simulink model "xieboduoji_13fangzhennow"  (R2023a)
settings: Solver=ode4  StartTime=0.0  StopTime=2.2  FixedStep=5e-7  RelTol=1e-3
undefined symbols (not defined in the file or in its folder): magnitude
libraries: simulink x417, spsRMSLib x70, spsCurrentMeasurementLib x32, spsVoltageMeasurementLib x31, powerlib_meascontrol x24, spsFourierLib x21, spsGroundLib x19, spsThreePhasePISectionLineLib x17, spsThreePhaseSeriesRLCBranchLib x14, spsdq0toAlphaBetaZeroLib x13, spsSeriesRLCBranchLib x11, spsUniversalBridgeLib x11
(part 8 of 12)

== system xieboduoji_13fangzhennow/node3/谐波源/Subsystem1/RMS1 ==
  u1 : Inport
  u3 : Inport  Port=2
  u4 : Inport  Port=3
  u5 : Inport  Port=4
  u6 : Inport  Port=5
  u2 : Inport  Port=6
  Trigger : TriggerPort  VariantControl=(inherit)
  Scope : Scope  Commented=on
  Scope1 : Scope  Commented=on
  xunidiandao : MATLAB Function  TreatAsAtomicUnit=on
  k1 : Outport  VectorParamsAs1DForOutWhenUnconnected=off
  k2 : Outport  Port=2  VectorParamsAs1DForOutWhenUnconnected=off
  k3 : Outport  Port=3  VectorParamsAs1DForOutWhenUnconnected=off
  k4 : Outport  Port=4  VectorParamsAs1DForOutWhenUnconnected=off
  k5 : Outport  Port=5  VectorParamsAs1DForOutWhenUnconnected=off
  k6 : Outport  Port=6  VectorParamsAs1DForOutWhenUnconnected=off
  k7 : Outport  Port=7  VectorParamsAs1DForOutWhenUnconnected=off
  k8 : Outport  Port=8  VectorParamsAs1DForOutWhenUnconnected=off
  k9 : Outport  Port=9  VectorParamsAs1DForOutWhenUnconnected=off
  k10 : Outport  Port=10  VectorParamsAs1DForOutWhenUnconnected=off
  k11 : Outport  Port=11  VectorParamsAs1DForOutWhenUnconnected=off
  k12 : Outport  Port=12  VectorParamsAs1DForOutWhenUnconnected=off
  wires:
  xunidiandao/13(x) -> Scope/1
  u3/1 -> xunidiandao/2(u2)
  u4/1 -> xunidiandao/3(u3)
  u5/1 -> xunidiandao/4(u4)
  u6/1 -> xunidiandao/5(u5)
  u2/1 -> xunidiandao/6(u6)
  u1/1 -> xunidiandao/1(u1)
  xunidiandao/12(y66) -> k12/1
  xunidiandao/11(y6) -> k11/1
  xunidiandao/10(y55) -> k10/1
  xunidiandao/9(y5) -> k9/1
  xunidiandao/8(y44) -> k8/1
  xunidiandao/7(y4) -> k7/1
  xunidiandao/6(y33) -> k6/1
  xunidiandao/5(y3) -> k5/1
  xunidiandao/4(y22) -> k4/1
  xunidiandao/3(y2) -> k3/1
  xunidiandao/2(y11) -> k2/1
  xunidiandao/1(y1) -> k1/1, Scope1/1

== system xieboduoji_13fangzhennow/node3/谐波源/Subsystem2/RMS1 ==
  u1 : Inport
  u3 : Inport  Port=2
  u4 : Inport  Port=3
  u5 : Inport  Port=4
  u6 : Inport  Port=5
  u2 : Inport  Port=6
  Trigger : TriggerPort  VariantControl=(inherit)
  Scope : Scope  Commented=on
  Scope1 : Scope  Commented=on
  xunidiandao : MATLAB Function  TreatAsAtomicUnit=on
  k1 : Outport  VectorParamsAs1DForOutWhenUnconnected=off
  k2 : Outport  Port=2  VectorParamsAs1DForOutWhenUnconnected=off
  k3 : Outport  Port=3  VectorParamsAs1DForOutWhenUnconnected=off
  k4 : Outport  Port=4  VectorParamsAs1DForOutWhenUnconnected=off
  k5 : Outport  Port=5  VectorParamsAs1DForOutWhenUnconnected=off
  k6 : Outport  Port=6  VectorParamsAs1DForOutWhenUnconnected=off
  k7 : Outport  Port=7  VectorParamsAs1DForOutWhenUnconnected=off
  k8 : Outport  Port=8  VectorParamsAs1DForOutWhenUnconnected=off
  k9 : Outport  Port=9  VectorParamsAs1DForOutWhenUnconnected=off
  k10 : Outport  Port=10  VectorParamsAs1DForOutWhenUnconnected=off
  k11 : Outport  Port=11  VectorParamsAs1DForOutWhenUnconnected=off
  k12 : Outport  Port=12  VectorParamsAs1DForOutWhenUnconnected=off
  wires:
  xunidiandao/1(y1) -> Scope1/1, k1/1
  xunidiandao/2(y11) -> k2/1
  xunidiandao/3(y2) -> k3/1
  xunidiandao/4(y22) -> k4/1
  xunidiandao/5(y3) -> k5/1
  xunidiandao/6(y33) -> k6/1
  xunidiandao/7(y4) -> k7/1
  xunidiandao/8(y44) -> k8/1
  xunidiandao/9(y5) -> k9/1
  xunidiandao/10(y55) -> k10/1
  xunidiandao/11(y6) -> k11/1
  xunidiandao/12(y66) -> k12/1
  u1/1 -> xunidiandao/1(u1)
  u2/1 -> xunidiandao/6(u6)
  u6/1 -> xunidiandao/5(u5)
  u5/1 -> xunidiandao/4(u4)
  u4/1 -> xunidiandao/3(u3)
  u3/1 -> xunidiandao/2(u2)
  xunidiandao/13(x) -> Scope/1

== system xieboduoji_13fangzhennow/node4/谐波源/Subsystem1/RMS1 ==
  u1 : Inport
  u3 : Inport  Port=2
  u4 : Inport  Port=3
  u5 : Inport  Port=4
  u6 : Inport  Port=5
  u2 : Inport  Port=6
  Trigger : TriggerPort  VariantControl=(inherit)
  Scope : Scope  Commented=on
  Scope1 : Scope  Commented=on
  xunidiandao : MATLAB Function  TreatAsAtomicUnit=on
  k1 : Outport  VectorParamsAs1DForOutWhenUnconnected=off
  k2 : Outport  Port=2  VectorParamsAs1DForOutWhenUnconnected=off
  k3 : Outport  Port=3  VectorParamsAs1DForOutWhenUnconnected=off
  k4 : Outport  Port=4  VectorParamsAs1DForOutWhenUnconnected=off
  k5 : Outport  Port=5  VectorParamsAs1DForOutWhenUnconnected=off
  k6 : Outport  Port=6  VectorParamsAs1DForOutWhenUnconnected=off
  k7 : Outport  Port=7  VectorParamsAs1DForOutWhenUnconnected=off
  k8 : Outport  Port=8  VectorParamsAs1DForOutWhenUnconnected=off
  k9 : Outport  Port=9  VectorParamsAs1DForOutWhenUnconnected=off
  k10 : Outport  Port=10  VectorParamsAs1DForOutWhenUnconnected=off
  k11 : Outport  Port=11  VectorParamsAs1DForOutWhenUnconnected=off
  k12 : Outport  Port=12  VectorParamsAs1DForOutWhenUnconnected=off
  wires:
  xunidiandao/13(x) -> Scope/1
  u3/1 -> xunidiandao/2(u2)
  u4/1 -> xunidiandao/3(u3)
  u5/1 -> xunidiandao/4(u4)
  u6/1 -> xunidiandao/5(u5)
  u2/1 -> xunidiandao/6(u6)
  u1/1 -> xunidiandao/1(u1)
  xunidiandao/12(y66) -> k12/1
  xunidiandao/11(y6) -> k11/1
  xunidiandao/10(y55) -> k10/1
  xunidiandao/9(y5) -> k9/1
  xunidiandao/8(y44) -> k8/1
  xunidiandao/7(y4) -> k7/1
  xunidiandao/6(y33) -> k6/1
  xunidiandao/5(y3) -> k5/1
  xunidiandao/4(y22) -> k4/1
  xunidiandao/3(y2) -> k3/1
  xunidiandao/2(y11) -> k2/1
  xunidiandao/1(y1) -> k1/1, Scope1/1

== system xieboduoji_13fangzhennow/node4/谐波源/Subsystem2/RMS1 ==
  u1 : Inport
  u3 : Inport  Port=2
  u4 : Inport  Port=3
  u5 : Inport  Port=4
  u6 : Inport  Port=5
  u2 : Inport  Port=6
  Trigger : TriggerPort  VariantControl=(inherit)
  Scope : Scope  Commented=on
  Scope1 : Scope  Commented=on
  xunidiandao : MATLAB Function  TreatAsAtomicUnit=on
  k1 : Outport  VectorParamsAs1DForOutWhenUnconnected=off
  k2 : Outport  Port=2  VectorParamsAs1DForOutWhenUnconnected=off
  k3 : Outport  Port=3  VectorParamsAs1DForOutWhenUnconnected=off
  k4 : Outport  Port=4  VectorParamsAs1DForOutWhenUnconnected=off
  k5 : Outport  Port=5  VectorParamsAs1DForOutWhenUnconnected=off
  k6 : Outport  Port=6  VectorParamsAs1DForOutWhenUnconnected=off
  k7 : Outport  Port=7  VectorParamsAs1DForOutWhenUnconnected=off
  k8 : Outport  Port=8  VectorParamsAs1DForOutWhenUnconnected=off
  k9 : Outport  Port=9  VectorParamsAs1DForOutWhenUnconnected=off
  k10 : Outport  Port=10  VectorParamsAs1DForOutWhenUnconnected=off
  k11 : Outport  Port=11  VectorParamsAs1DForOutWhenUnconnected=off
  k12 : Outport  Port=12  VectorParamsAs1DForOutWhenUnconnected=off
  wires:
  xunidiandao/1(y1) -> Scope1/1, k1/1
  xunidiandao/2(y11) -> k2/1
  xunidiandao/3(y2) -> k3/1
  xunidiandao/4(y22) -> k4/1
  xunidiandao/5(y3) -> k5/1
  xunidiandao/6(y33) -> k6/1
  xunidiandao/7(y4) -> k7/1
  xunidiandao/8(y44) -> k8/1
  xunidiandao/9(y5) -> k9/1
  xunidiandao/10(y55) -> k10/1
  xunidiandao/11(y6) -> k11/1
  xunidiandao/12(y66) -> k12/1
  u1/1 -> xunidiandao/1(u1)
  u2/1 -> xunidiandao/6(u6)
  u6/1 -> xunidiandao/5(u5)
  u5/1 -> xunidiandao/4(u4)
  u4/1 -> xunidiandao/3(u3)
  u3/1 -> xunidiandao/2(u2)
  xunidiandao/13(x) -> Scope/1

== system xieboduoji_13fangzhennow/node5/谐波源/Subsystem1/RMS1 ==
  u1 : Inport
  u3 : Inport  Port=2
  u4 : Inport  Port=3
  u5 : Inport  Port=4
  u6 : Inport  Port=5
  u2 : Inport  Port=6
  Trigger : TriggerPort  VariantControl=(inherit)
  Scope : Scope  Commented=on
  Scope1 : Scope  Commented=on
  xunidiandao : MATLAB Function  TreatAsAtomicUnit=on
  k1 : Outport  VectorParamsAs1DForOutWhenUnconnected=off
  k2 : Outport  Port=2  VectorParamsAs1DForOutWhenUnconnected=off
  k3 : Outport  Port=3  VectorParamsAs1DForOutWhenUnconnected=off
  k4 : Outport  Port=4  VectorParamsAs1DForOutWhenUnconnected=off
  k5 : Outport  Port=5  VectorParamsAs1DForOutWhenUnconnected=off
  k6 : Outport  Port=6  VectorParamsAs1DForOutWhenUnconnected=off
  k7 : Outport  Port=7  VectorParamsAs1DForOutWhenUnconnected=off
  k8 : Outport  Port=8  VectorParamsAs1DForOutWhenUnconnected=off
  k9 : Outport  Port=9  VectorParamsAs1DForOutWhenUnconnected=off
  k10 : Outport  Port=10  VectorParamsAs1DForOutWhenUnconnected=off
  k11 : Outport  Port=11  VectorParamsAs1DForOutWhenUnconnected=off
  k12 : Outport  Port=12  VectorParamsAs1DForOutWhenUnconnected=off
  wires:
  xunidiandao/13(x) -> Scope/1
  u3/1 -> xunidiandao/2(u2)
  u4/1 -> xunidiandao/3(u3)
  u5/1 -> xunidiandao/4(u4)
  u6/1 -> xunidiandao/5(u5)
  u2/1 -> xunidiandao/6(u6)
  u1/1 -> xunidiandao/1(u1)
  xunidiandao/12(y66) -> k12/1
  xunidiandao/11(y6) -> k11/1
  xunidiandao/10(y55) -> k10/1
  xunidiandao/9(y5) -> k9/1
  xunidiandao/8(y44) -> k8/1
  xunidiandao/7(y4) -> k7/1
  xunidiandao/6(y33) -> k6/1
  xunidiandao/5(y3) -> k5/1
  xunidiandao/4(y22) -> k4/1
  xunidiandao/3(y2) -> k3/1
  xunidiandao/2(y11) -> k2/1
  xunidiandao/1(y1) -> k1/1, Scope1/1

== system xieboduoji_13fangzhennow/node5/谐波源/Subsystem2/RMS1 ==
  u1 : Inport
  u3 : Inport  Port=2
  u4 : Inport  Port=3
  u5 : Inport  Port=4
  u6 : Inport  Port=5
  u2 : Inport  Port=6
  Trigger : TriggerPort  VariantControl=(inherit)
  Scope : Scope  Commented=on
  Scope1 : Scope  Commented=on
  xunidiandao : MATLAB Function  TreatAsAtomicUnit=on
  k1 : Outport  VectorParamsAs1DForOutWhenUnconnected=off
  k2 : Outport  Port=2  VectorParamsAs1DForOutWhenUnconnected=off
  k3 : Outport  Port=3  VectorParamsAs1DForOutWhenUnconnected=off
  k4 : Outport  Port=4  VectorParamsAs1DForOutWhenUnconnected=off
  k5 : Outport  Port=5  VectorParamsAs1DForOutWhenUnconnected=off
  k6 : Outport  Port=6  VectorParamsAs1DForOutWhenUnconnected=off
  k7 : Outport  Port=7  VectorParamsAs1DForOutWhenUnconnected=off
  k8 : Outport  Port=8  VectorParamsAs1DForOutWhenUnconnected=off
  k9 : Outport  Port=9  VectorParamsAs1DForOutWhenUnconnected=off
  k10 : Outport  Port=10  VectorParamsAs1DForOutWhenUnconnected=off
  k11 : Outport  Port=11  VectorParamsAs1DForOutWhenUnconnected=off
  k12 : Outport  Port=12  VectorParamsAs1DForOutWhenUnconnected=off
  wires:
  xunidiandao/1(y1) -> Scope1/1, k1/1
  xunidiandao/2(y11) -> k2/1
  xunidiandao/3(y2) -> k3/1
  xunidiandao/4(y22) -> k4/1
  xunidiandao/5(y3) -> k5/1
  xunidiandao/6(y33) -> k6/1
  xunidiandao/7(y4) -> k7/1
  xunidiandao/8(y44) -> k8/1
  xunidiandao/9(y5) -> k9/1
  xunidiandao/10(y55) -> k10/1
  xunidiandao/11(y6) -> k11/1
  xunidiandao/12(y66) -> k12/1
  u1/1 -> xunidiandao/1(u1)
  u2/1 -> xunidiandao/6(u6)
  u6/1 -> xunidiandao/5(u5)
  u5/1 -> xunidiandao/4(u4)
  u4/1 -> xunidiandao/3(u3)
  u3/1 -> xunidiandao/2(u2)
  xunidiandao/13(x) -> Scope/1

== system xieboduoji_13fangzhennow/node8/谐波源/Subsystem1/RMS1 ==
  u1 : Inport
  u3 : Inport  Port=2
  u4 : Inport  Port=3
  u5 : Inport  Port=4
  u6 : Inport  Port=5
  u2 : Inport  Port=6
  Trigger : TriggerPort  VariantControl=(inherit)
  Scope : Scope  Commented=on
  Scope1 : Scope  Commented=on
  xunidiandao : MATLAB Function  TreatAsAtomicUnit=on
  k1 : Outport  VectorParamsAs1DForOutWhenUnconnected=off
  k2 : Outport  Port=2  VectorParamsAs1DForOutWhenUnconnected=off
  k3 : Outport  Port=3  VectorParamsAs1DForOutWhenUnconnected=off
  k4 : Outport  Port=4  VectorParamsAs1DForOutWhenUnconnected=off
  k5 : Outport  Port=5  VectorParamsAs1DForOutWhenUnconnected=off
  k6 : Outport  Port=6  VectorParamsAs1DForOutWhenUnconnected=off
  k7 : Outport  Port=7  VectorParamsAs1DForOutWhenUnconnected=off
  k8 : Outport  Port=8  VectorParamsAs1DForOutWhenUnconnected=off
  k9 : Outport  Port=9  VectorParamsAs1DForOutWhenUnconnected=off
  k10 : Outport  Port=10  VectorParamsAs1DForOutWhenUnconnected=off
  k11 : Outport  Port=11  VectorParamsAs1DForOutWhenUnconnected=off
  k12 : Outport  Port=12  VectorParamsAs1DForOutWhenUnconnected=off
  wires:
  xunidiandao/13(x) -> Scope/1
  u3/1 -> xunidiandao/2(u2)
  u4/1 -> xunidiandao/3(u3)
  u5/1 -> xunidiandao/4(u4)
  u6/1 -> xunidiandao/5(u5)
  u2/1 -> xunidiandao/6(u6)
  u1/1 -> xunidiandao/1(u1)
  xunidiandao/12(y66) -> k12/1
  xunidiandao/11(y6) -> k11/1
  xunidiandao/10(y55) -> k10/1
  xunidiandao/9(y5) -> k9/1
  xunidiandao/8(y44) -> k8/1
  xunidiandao/7(y4) -> k7/1
  xunidiandao/6(y33) -> k6/1
  xunidiandao/5(y3) -> k5/1
  xunidiandao/4(y22) -> k4/1
  xunidiandao/3(y2) -> k3/1
  xunidiandao/2(y11) -> k2/1
  xunidiandao/1(y1) -> k1/1, Scope1/1

== system xieboduoji_13fangzhennow/node8/谐波源/Subsystem2/RMS1 ==
  u1 : Inport
  u3 : Inport  Port=2
  u4 : Inport  Port=3
  u5 : Inport  Port=4
  u6 : Inport  Port=5
  u2 : Inport  Port=6
  Trigger : TriggerPort  VariantControl=(inherit)
  Scope : Scope  Commented=on
  Scope1 : Scope  Commented=on
  xunidiandao : MATLAB Function  TreatAsAtomicUnit=on
  k1 : Outport  VectorParamsAs1DForOutWhenUnconnected=off
  k2 : Outport  Port=2  VectorParamsAs1DForOutWhenUnconnected=off
  k3 : Outport  Port=3  VectorParamsAs1DForOutWhenUnconnected=off
  k4 : Outport  Port=4  VectorParamsAs1DForOutWhenUnconnected=off
  k5 : Outport  Port=5  VectorParamsAs1DForOutWhenUnconnected=off
  k6 : Outport  Port=6  VectorParamsAs1DForOutWhenUnconnected=off
  k7 : Outport  Port=7  VectorParamsAs1DForOutWhenUnconnected=off
  k8 : Outport  Port=8  VectorParamsAs1DForOutWhenUnconnected=off
  k9 : Outport  Port=9  VectorParamsAs1DForOutWhenUnconnected=off
  k10 : Outport  Port=10  VectorParamsAs1DForOutWhenUnconnected=off
  k11 : Outport  Port=11  VectorParamsAs1DForOutWhenUnconnected=off
  k12 : Outport  Port=12  VectorParamsAs1DForOutWhenUnconnected=off
  wires:
  xunidiandao/1(y1) -> Scope1/1, k1/1
  xunidiandao/2(y11) -> k2/1
  xunidiandao/3(y2) -> k3/1
  xunidiandao/4(y22) -> k4/1
  xunidiandao/5(y3) -> k5/1
  xunidiandao/6(y33) -> k6/1
  xunidiandao/7(y4) -> k7/1
  xunidiandao/8(y44) -> k8/1
  xunidiandao/9(y5) -> k9/1
  xunidiandao/10(y55) -> k10/1
  xunidiandao/11(y6) -> k11/1
  xunidiandao/12(y66) -> k12/1
  u1/1 -> xunidiandao/1(u1)
  u2/1 -> xunidiandao/6(u6)
  u6/1 -> xunidiandao/5(u5)
  u5/1 -> xunidiandao/4(u4)
  u4/1 -> xunidiandao/3(u3)
  u3/1 -> xunidiandao/2(u2)
  xunidiandao/13(x) -> Scope/1

== system xieboduoji_13fangzhennow/node12/PV15kW3/谐波检测/Subsystem/Sub ==
  In1 : Inport
  Constant1 : Constant  Value=-60*pi/180
  Constant{10,12,15,17} (4 alike) : Constant  Value=100*pi
  Constant11 : Constant  Value=5
  Constant2 : Constant  Value=-60*pi/180
  Cos : Trigonometry  Operator=cos
  Cos1 : Trigonometry  Operator=cos
  Cos2 : Trigonometry
  Cos3 : Trigonometry
  Delay : Delay  DelayLength=400  SampleTime=5e-5
  Delay1 : Delay  DelayLength=1  SampleTime=5e-5
  Delay2 : Delay  DelayLength=1  SampleTime=5e-5
  Divide{,1..3} (4 alike) : Product  Inputs=***
  Dot Product{,1..2,4} (4 alike) : DotProduct  OutDataTypeStr=Inherit: Inherit via internal rule
  Gain : Gain  Gain=2/400
  Gain10 : Gain  Gain=2/400
  Ramp{,1..3} (4 alike) : simulink/Sources/Ramp  slope=1  start=0  InitialOutput=0
  Sum{,1,3,9,18} (5 alike) : Sum  Inputs=|++
  Sum2 : Sum  Inputs=-+|
  u1 : Outport
  wires:
  [thk] -> Divide/1
  Constant11/1 -> [thk]
  Sum9/1 -> u1/1
  Dot Product1/1 -> Sum9/1
  Gain/1 -> Sum3/1
  Ramp2/1 -> Divide2/3
  Constant10/1 -> Divide/2
  Delay2/1 -> Sum18/2
  Gain10/1 -> Sum18/1
  Sum3/1 -> Delay1/1, Dot Product1/2
  Delay/1 -> Sum2/1
  Ramp1/1 -> Divide1/3
  Constant12/1 -> Divide1/2
  Divide2/1 -> Cos2/1
  Cos3/1 -> Dot Product4/2
  Dot Product2/1 -> Gain10/1
  Cos2/1 -> Dot Product2/2
  Delay1/1 -> Sum3/2
  Ramp3/1 -> Divide3/3
  [thk] -> Divide1/1
  Dot Product4/1 -> Sum9/2
  [thk] -> Divide2/1
  [thk] -> Divide3/1
  Sum18/1 -> Delay2/1, Dot Product4/1
  Constant15/1 -> Divide2/2
  In1/1 -> Sum2/2, Delay/1
  Dot Product/1 -> Gain/1
  Cos/1 -> Dot Product/1
  Divide/1 -> Cos/1
  Sum2/1 -> Dot Product/2, Dot Product2/1
  Ramp/1 -> Divide/3
  Constant17/1 -> Divide3/2
  Cos1/1 -> Dot Product1/1
  Divide1/1 -> Sum/1
  Sum/1 -> Cos1/1
  Sum1/1 -> Cos3/1
  Divide3/1 -> Sum1/1

== system xieboduoji_13fangzhennow/node12/PV15kW3/谐波检测/Subsystem/Sub1 ==
  In1 : Inport
  Constant1 : Constant  Value=-60*pi/180
  Constant{10,12,15,17} (4 alike) : Constant  Value=100*pi
  Constant11 : Constant  Value=7
  Constant2 : Constant  Value=-60*pi/180
  Cos : Trigonometry  Operator=cos
  Cos1 : Trigonometry  Operator=cos
  Cos2 : Trigonometry
  Cos3 : Trigonometry
  Delay : Delay  DelayLength=400  SampleTime=5e-5
  Delay1 : Delay  DelayLength=1  SampleTime=5e-5
  Delay2 : Delay  DelayLength=1  SampleTime=5e-5
  Divide{,1..3} (4 alike) : Product  Inputs=***
  Dot Product{,1..2,4} (4 alike) : DotProduct  OutDataTypeStr=Inherit: Inherit via internal rule
  Gain : Gain  Gain=2/400
  Gain10 : Gain  Gain=2/400
  Ramp{,1..3} (4 alike) : simulink/Sources/Ramp  slope=1  start=0  InitialOutput=0
  Sum{,1,3,9,18} (5 alike) : Sum  Inputs=|++
  Sum2 : Sum  Inputs=-+|
  u1 : Outport
  wires:
  Divide3/1 -> Sum1/1
  Sum1/1 -> Cos3/1
  Sum/1 -> Cos1/1
  Divide1/1 -> Sum/1
  Cos1/1 -> Dot Product1/1
  Constant17/1 -> Divide3/2
  Ramp/1 -> Divide/3
  Sum2/1 -> Dot Product2/1, Dot Product/2
  Divide/1 -> Cos/1
  Cos/1 -> Dot Product/1
  Dot Product/1 -> Gain/1
  In1/1 -> Delay/1, Sum2/2
  Constant15/1 -> Divide2/2
  Sum18/1 -> Dot Product4/1, Delay2/1
  [thk] -> Divide3/1
  [thk] -> Divide2/1
  Dot Product4/1 -> Sum9/2
  [thk] -> Divide1/1
  Ramp3/1 -> Divide3/3
  Delay1/1 -> Sum3/2
  Cos2/1 -> Dot Product2/2
  Dot Product2/1 -> Gain10/1
  Cos3/1 -> Dot Product4/2
  Divide2/1 -> Cos2/1
  Constant12/1 -> Divide1/2
  Ramp1/1 -> Divide1/3
  Delay/1 -> Sum2/1
  Sum3/1 -> Dot Product1/2, Delay1/1
  Gain10/1 -> Sum18/1
  Delay2/1 -> Sum18/2
  Constant10/1 -> Divide/2
  Ramp2/1 -> Divide2/3
  Gain/1 -> Sum3/1
  Dot Product1/1 -> Sum9/1
  Sum9/1 -> u1/1
  Constant11/1 -> [thk]
  [thk] -> Divide/1

== system xieboduoji_13fangzhennow/node12/PV15kW3/谐波检测/Subsystem/Sub10 ==
  In1 : Inport
  Constant1 : Constant  Value=10*pi/180
  Constant{10,12,15,17} (4 alike) : Constant  Value=100*pi
  Constant11 : Constant  Value=19
  Constant2 : Constant  Value=10*pi/180
  Cos : Trigonometry  Operator=cos
  Cos1 : Trigonometry  Operator=cos
  Cos2 : Trigonometry
  Cos3 : Trigonometry
  Delay : Delay  DelayLength=400  SampleTime=5e-5
  Delay1 : Delay  DelayLength=1  SampleTime=5e-5
  Delay2 : Delay  DelayLength=1  SampleTime=5e-5
  Divide{,1..3} (4 alike) : Product  Inputs=***
  Dot Product{,1..2,4} (4 alike) : DotProduct  OutDataTypeStr=Inherit: Inherit via internal rule
  Gain : Gain  Gain=2/400
  Gain10 : Gain  Gain=2/400
  Ramp{,1..3} (4 alike) : simulink/Sources/Ramp  slope=1  start=0  InitialOutput=0
  Sum{,1,3,9,18} (5 alike) : Sum  Inputs=|++
  Sum2 : Sum  Inputs=-+|
  u9 : Outport
  wires:
  [thk] -> Divide/1
  Constant11/1 -> [thk]
  Sum9/1 -> u9/1
  Dot Product1/1 -> Sum9/1
  Gain/1 -> Sum3/1
  Ramp2/1 -> Divide2/3
  Constant10/1 -> Divide/2
  Delay2/1 -> Sum18/2
  Gain10/1 -> Sum18/1
  Sum3/1 -> Delay1/1, Dot Product1/2
  Delay/1 -> Sum2/1
  Ramp1/1 -> Divide1/3
  Constant12/1 -> Divide1/2
  Divide2/1 -> Cos2/1
  Cos3/1 -> Dot Product4/2
  Dot Product2/1 -> Gain10/1
  Cos2/1 -> Dot Product2/2
  Delay1/1 -> Sum3/2
  Ramp3/1 -> Divide3/3
  [thk] -> Divide1/1
  Dot Product4/1 -> Sum9/2
  [thk] -> Divide2/1
  [thk] -> Divide3/1
  Sum18/1 -> Delay2/1, Dot Product4/1
  Constant15/1 -> Divide2/2
  In1/1 -> Sum2/2, Delay/1
  Cos1/1 -> Dot Product1/1
  Dot Product/1 -> Gain/1
  Cos/1 -> Dot Product/1
  Divide/1 -> Cos/1
  Sum2/1 -> Dot Product/2, Dot Product2/1
  Ramp/1 -> Divide/3
  Constant17/1 -> Divide3/2
  Divide1/1 -> Sum/1
  Sum/1 -> Cos1/1
  Divide3/1 -> Sum1/1
  Sum1/1 -> Cos3/1
  Constant2/1 -> Sum/2
  Constant1/1 -> Sum1/2

== system xieboduoji_13fangzhennow/node12/PV15kW3/谐波检测/Subsystem/Sub12 ==
  In1 : Inport
  Constant1 : Constant  Value=10*pi/180
  Constant{10,12,15,17} (4 alike) : Constant  Value=100*pi
  Constant11 : Constant  Value=17
  Constant2 : Constant  Value=10*pi/180
  Cos : Trigonometry  Operator=cos
  Cos1 : Trigonometry  Operator=cos
  Cos2 : Trigonometry
  Cos3 : Trigonometry
  Delay : Delay  DelayLength=400  SampleTime=5e-5
  Delay1 : Delay  DelayLength=1  SampleTime=5e-5
  Delay2 : Delay  DelayLength=1  SampleTime=5e-5
  Divide{,1..3} (4 alike) : Product  Inputs=***
  Dot Product{,1..2,4} (4 alike) : DotProduct  OutDataTypeStr=Inherit: Inherit via internal rule
  Gain : Gain  Gain=2/400
  Gain10 : Gain  Gain=2/400
  Ramp{,1..3} (4 alike) : simulink/Sources/Ramp  slope=1  start=0  InitialOutput=0
  Sum{,1,3,9,18} (5 alike) : Sum  Inputs=|++
  Sum2 : Sum  Inputs=-+|
  u9 : Outport
  wires:
  Constant1/1 -> Sum1/2
  Constant2/1 -> Sum/2
  Sum1/1 -> Cos3/1
  Divide3/1 -> Sum1/1
  Sum/1 -> Cos1/1
  Divide1/1 -> Sum/1
  Constant17/1 -> Divide3/2
  Ramp/1 -> Divide/3
  Sum2/1 -> Dot Product2/1, Dot Product/2
  Divide/1 -> Cos/1
  Cos/1 -> Dot Product/1
  Dot Product/1 -> Gain/1
  Cos1/1 -> Dot Product1/1
  In1/1 -> Delay/1, Sum2/2
  Constant15/1 -> Divide2/2
  Sum18/1 -> Dot Product4/1, Delay2/1
  [thk] -> Divide3/1
  [thk] -> Divide2/1
  Dot Product4/1 -> Sum9/2
  [thk] -> Divide1/1
  Ramp3/1 -> Divide3/3
  Delay1/1 -> Sum3/2
  Cos2/1 -> Dot Product2/2
  Dot Product2/1 -> Gain10/1
  Cos3/1 -> Dot Product4/2
  Divide2/1 -> Cos2/1
  Constant12/1 -> Divide1/2
  Ramp1/1 -> Divide1/3
  Delay/1 -> Sum2/1
  Sum3/1 -> Dot Product1/2, Delay1/1
  Gain10/1 -> Sum18/1
  Delay2/1 -> Sum18/2
  Constant10/1 -> Divide/2
  Ramp2/1 -> Divide2/3
  Gain/1 -> Sum3/1
  Dot Product1/1 -> Sum9/1
  Sum9/1 -> u9/1
  Constant11/1 -> [thk]
  [thk] -> Divide/1

== system xieboduoji_13fangzhennow/node12/PV15kW3/谐波检测/Subsystem/Sub2 ==
  In1 : Inport
  Constant1 : Constant  Value=-15*pi/180
  Constant{10,12,15,17} (4 alike) : Constant  Value=100*pi
  Constant11 : Constant  Value=11
  Constant2 : Constant  Value=-15*pi/180
  Cos : Trigonometry  Operator=cos
  Cos2 : Trigonometry
  Cos3 : Trigonometry
  Cos4 : Trigonometry  Operator=cos
  Delay : Delay  DelayLength=400  SampleTime=5e-5
  Delay1 : Delay  DelayLength=1  SampleTime=5e-5
  Delay2 : Delay  DelayLength=1  SampleTime=5e-5
  Divide{,1..3} (4 alike) : Product  Inputs=***
  Dot Product{,1..2,4} (4 alike) : DotProduct  OutDataTypeStr=Inherit: Inherit via internal rule
  Gain : Gain  Gain=2/400
  Gain10 : Gain  Gain=2/400
  Ramp{,1..3} (4 alike) : simulink/Sources/Ramp  slope=1  start=0  InitialOutput=0
  Sum{,1,3,9,18} (5 alike) : Sum  Inputs=|++
  Sum2 : Sum  Inputs=-+|
  u5 : Outport
  wires:
  [thk] -> Divide/1
  Constant11/1 -> [thk]
  Sum9/1 -> u5/1
  Dot Product1/1 -> Sum9/1
  Gain/1 -> Sum3/1
  Ramp2/1 -> Divide2/3
  Constant10/1 -> Divide/2
  Delay2/1 -> Sum18/2
  Gain10/1 -> Sum18/1
  Sum3/1 -> Delay1/1, Dot Product1/2
  Delay/1 -> Sum2/1
  Ramp1/1 -> Divide1/3
  Constant12/1 -> Divide1/2
  Divide2/1 -> Cos2/1
  Cos3/1 -> Dot Product4/2
  Dot Product2/1 -> Gain10/1
  Cos2/1 -> Dot Product2/2
  Delay1/1 -> Sum3/2
  Ramp3/1 -> Divide3/3
  [thk] -> Divide1/1
  Dot Product4/1 -> Sum9/2
  [thk] -> Divide2/1
  [thk] -> Divide3/1
  Sum18/1 -> Delay2/1, Dot Product4/1
  Constant15/1 -> Divide2/2
  In1/1 -> Sum2/2, Delay/1
  Dot Product/1 -> Gain/1
  Cos/1 -> Dot Product/1
  Divide/1 -> Cos/1
  Sum2/1 -> Dot Product/2, Dot Product2/1
  Ramp/1 -> Divide/3
  Constant17/1 -> Divide3/2
  Divide1/1 -> Sum/1
  Constant2/1 -> Sum/2
  Sum/1 -> Cos4/1
  Cos4/1 -> Dot Product1/1
  Divide3/1 -> Sum1/1
  Constant1/1 -> Sum1/2
  Sum1/1 -> Cos3/1

== system xieboduoji_13fangzhennow/node12/PV15kW3/谐波检测/Subsystem/Sub3 ==
  In1 : Inport
  Constant1 : Constant  Value=-15*pi/180
  Constant{10,12,15,17} (4 alike) : Constant  Value=100*pi
  Constant11 : Constant  Value=13
  Constant2 : Constant  Value=-15*pi/180
  Cos : Trigonometry  Operator=cos
  Cos1 : Trigonometry  Operator=cos
  Cos2 : Trigonometry
  Cos3 : Trigonometry
  Delay : Delay  DelayLength=400  SampleTime=5e-5
  Delay1 : Delay  DelayLength=1  SampleTime=5e-5
  Delay2 : Delay  DelayLength=1  SampleTime=5e-5
  Divide{,1..3} (4 alike) : Product  Inputs=***
  Dot Product{,1..2,4} (4 alike) : DotProduct  OutDataTypeStr=Inherit: Inherit via internal rule
  Gain : Gain  Gain=2/400
  Gain10 : Gain  Gain=2/400
  Ramp{,1..3} (4 alike) : simulink/Sources/Ramp  slope=1  start=0  InitialOutput=0
  Sum{,1,3,9,18} (5 alike) : Sum  Inputs=|++
  Sum2 : Sum  Inputs=-+|
  u7 : Outport
  wires:
  Constant17/1 -> Divide3/2
  Ramp/1 -> Divide/3
  Sum2/1 -> Dot Product2/1, Dot Product/2
  Divide/1 -> Cos/1
  Cos/1 -> Dot Product/1
  Dot Product/1 -> Gain/1
  Cos1/1 -> Dot Product1/1
  In1/1 -> Delay/1, Sum2/2
  Constant15/1 -> Divide2/2
  Sum18/1 -> Dot Product4/1, Delay2/1
  [thk] -> Divide3/1
  [thk] -> Divide2/1
  Dot Product4/1 -> Sum9/2
  [thk] -> Divide1/1
  Ramp3/1 -> Divide3/3
  Delay1/1 -> Sum3/2
  Cos2/1 -> Dot Product2/2
  Dot Product2/1 -> Gain10/1
  Cos3/1 -> Dot Product4/2
  Divide2/1 -> Cos2/1
  Constant12/1 -> Divide1/2
  Ramp1/1 -> Divide1/3
  Delay/1 -> Sum2/1
  Sum3/1 -> Dot Product1/2, Delay1/1
  Gain10/1 -> Sum18/1
  Delay2/1 -> Sum18/2
  Constant10/1 -> Divide/2
  Ramp2/1 -> Divide2/3
  Gain/1 -> Sum3/1
  Dot Product1/1 -> Sum9/1
  Sum9/1 -> u7/1
  Constant11/1 -> [thk]
  [thk] -> Divide/1
  Divide1/1 -> Sum/1
  Constant2/1 -> Sum/2
  Sum/1 -> Cos1/1
  Divide3/1 -> Sum1/1
  Constant1/1 -> Sum1/2
  Sum1/1 -> Cos3/1

== system xieboduoji_13fangzhennow/node12/PV15kW3/谐波检测/Subsystem/Sub4 ==
  In1 : Inport
  Constant1 : Constant  Value=10*pi/180
  Constant{10,12,15,17} (4 alike) : Constant  Value=100*pi
  Constant11 : Constant  Value=17
  Constant2 : Constant  Value=10*pi/180
  Cos : Trigonometry  Operator=cos
  Cos1 : Trigonometry  Operator=cos
  Cos2 : Trigonometry
  Cos3 : Trigonometry
  Delay : Delay  DelayLength=400  SampleTime=5e-5
  Delay1 : Delay  DelayLength=1  SampleTime=5e-5
  Delay2 : Delay  DelayLength=1  SampleTime=5e-5
  Divide{,1..3} (4 alike) : Product  Inputs=***
  Dot Product{,1..2,4} (4 alike) : DotProduct  OutDataTypeStr=Inherit: Inherit via internal rule
  Gain : Gain  Gain=2/400
  Gain10 : Gain  Gain=2/400
  Ramp{,1..3} (4 alike) : simulink/Sources/Ramp  slope=1  start=0  InitialOutput=0
  Sum{,1,3,9,18} (5 alike) : Sum  Inputs=|++
  Sum2 : Sum  Inputs=-+|
  u9 : Outport
  wires:
  [thk] -> Divide/1
  Constant11/1 -> [thk]
  Sum9/1 -> u9/1
  Dot Product1/1 -> Sum9/1
  Gain/1 -> Sum3/1
  Ramp2/1 -> Divide2/3
  Constant10/1 -> Divide/2
  Delay2/1 -> Sum18/2
  Gain10/1 -> Sum18/1
  Sum3/1 -> Delay1/1, Dot Product1/2
  Delay/1 -> Sum2/1
  Ramp1/1 -> Divide1/3
  Constant12/1 -> Divide1/2
  Divide2/1 -> Cos2/1
  Cos3/1 -> Dot Product4/2
  Dot Product2/1 -> Gain10/1
  Cos2/1 -> Dot Product2/2
  Delay1/1 -> Sum3/2
  Ramp3/1 -> Divide3/3
  [thk] -> Divide1/1
  Dot Product4/1 -> Sum9/2
  [thk] -> Divide2/1
  [thk] -> Divide3/1
  Sum18/1 -> Delay2/1, Dot Product4/1
  Constant15/1 -> Divide2/2
  In1/1 -> Sum2/2, Delay/1
  Cos1/1 -> Dot Product1/1
  Dot Product/1 -> Gain/1
  Cos/1 -> Dot Product/1
  Divide/1 -> Cos/1
  Sum2/1 -> Dot Product/2, Dot Product2/1
  Ramp/1 -> Divide/3
  Constant17/1 -> Divide3/2
  Divide1/1 -> Sum/1
  Sum/1 -> Cos1/1
  Divide3/1 -> Sum1/1
  Sum1/1 -> Cos3/1
  Constant2/1 -> Sum/2
  Constant1/1 -> Sum1/2

== system xieboduoji_13fangzhennow/node12/PV15kW3/谐波检测/Subsystem/Sub5 ==
  In1 : Inport
  Add : Sum
  Constant1 : Constant  Value=10*pi/180
  Constant{10,12,15,17} (4 alike) : Constant  Value=100*pi
  Constant11 : Constant  Value=19
  Constant2 : Constant  Value=10*pi/180
  Cos : Trigonometry  Operator=cos
  Cos1 : Trigonometry  Operator=cos
  Cos2 : Trigonometry
  Cos3 : Trigonometry
  Delay : Delay  DelayLength=400  SampleTime=5e-5
  Delay1 : Delay  DelayLength=1  SampleTime=5e-5
  Delay2 : Delay  DelayLength=1  SampleTime=5e-5
  Discrete PID Controller : slpidlib/PID Controller  Controller=P  Form=Parallel  TimeDomain=Discrete-time  UseExternalTs=off  SampleTime=5e-5  IntegratorMethod=Forward Euler  FilterMethod=Forward Euler  ControllerParametersSource=internal  P=1  I=1  UseKiTs=off  D=0  N=100  UseFilter=on  TunerSelectOption=Transfer Function Based (PID Tuner App)  InitialConditionSource=internal  InitialConditionForIntegrator=0  InitialConditionForFilter=0  DifferentiatorICPrevScaledInput=0  ExternalReset=none  TrackingMode=off  Kt=1  LimitOutput=off  SatLimitsSource=internal  UpperSaturationLimit=inf  LowerSaturationLimit=-inf  LinearizeAsGain=off  AntiWindupMode=none  Kb=1  LimitIntegrator=off  UpperIntegratorSaturationLimit=inf  LowerIntegratorSaturationLimit=-inf  POutMin=[]  POutMax=[]  IOutMin=[]  IOutMax=[]  DOutMin=[]  DOutMax=[]  NOutMin=[]  NOutMax=[]  SumOutMin=[]  SumOutMax=[]  SaturationOutMin=[]  SaturationOutMax=[]  PParamMin=[]  PParamMax=[]  IParamMin=[]  IParamMax=[]  DParamMin=[]  DParamMax=[]  NParamMin=[]  NParamMax=[]  KbParamMin=[]  KbParamMax=[]  KtParamMin=[]  KtParamMax=[]  KbOutMin=[]  KbOutMax=[]  KtOutMin=[]  KtOutMax=[]  IntegratorOutMin=[]  IntegratorOutMax=[]  FilterOutMin=[]  FilterOutMax=[]  SumI1OutMin=[]  SumI1OutMax=[]  SumI2OutMin=[]  SumI2OutMax=[]  SumI3OutMin=[]  SumI3OutMax=[]  SumI4OutMin=[]  SumI4OutMax=[]  SumDOutMin=[]  SumDOutMax=[]  DifferentiatorOutMin=[]  DifferentiatorOutMax=[]  FilterDiffOutCoefMin=[]  FilterDiffOutCoefMax=[]  ReciprocalOutMin=[]  ReciprocalOutMax=[]  SumDenOutMin=[]  SumDenOutMax=[]  SumNumOutMin=[]  SumNumOutMax=[]  DivideOutMin=[]  DivideOutMax=[]  UdiffTsProdOutMin=[]  UdiffTsProdOutMax=[]  NTsProdOutMin=[]  NTsProdOutMax=[]  UintegralTsProdOutMin=[]  UintegralTsProdOutMax=[]  UngainTsProdOutMin=[]  UngainTsProdOutMax=[]  ClampingZeroOutDataTypeStr=Inherit: Inherit via back propagation  ClampingZeroOutMin=[]  ClampingZeroOutMax=[]  FilterDenConstantOutDataTypeStr=Inherit: Inherit via back propagation  FilterDenConstantOutMin=[]  FilterDenConstantOutMax=[]  PCopyOutDataTypeStr=Inherit: Inherit via back propagation  PCopyOutMin=[]  PCopyOutMax=[]  NCopyOutDataTypeStr=Inherit: Inherit via back propagation  NCopyOutMin=[]  NCopyOutMax=[]  IntegratorContinuousStateAttributes=''  IntegratorStateMustResolveToSignalObject=off  IntegratorRTWStateStorageClass=Auto  FilterContinuousStateAttributes=''  FilterStateMustResolveToSignalObject=off  FilterRTWStateStorageClass=Auto  ParallelPVariant=InternalParameters  IdealPVariant=Disabled  IVariant=Disabled  DVariant=Disabled  IntegratorVariant=Disabled  SatVariant=Disabled  AWVariant=Disabled  PCopyVariant=Disabled  TRVariant=Disabled  FdbkBlocksVariant=Forward  IdealPFdbkVariant=Disabled  SatFdbkVariant=Disabled  DerivativeFilterVariant=Disabled  NVariant=Disabled  NCopyVariant=Disabled_SignalSpec  FilterICVariant=Disabled  IntegratorICVariant=Disabled  ExternalResetVariant=Disabled  TRSumVariant=Passthrough  SumFdbkVariant=Disabled  SumVariant=Passthrough_P  TsampFilterVariant=InternalTs  TsampNgainVariant=Passthrough  TsampIntegralVariant=Disabled_SignalSpec  ExternalSaturationOutDataTypeStr=Inherit: Same as second input
  Discrete PID Controller1 : slpidlib/PID Controller  Controller=P  Form=Parallel  TimeDomain=Discrete-time  UseExternalTs=off  SampleTime=5e-5  IntegratorMethod=Forward Euler  FilterMethod=Forward Euler  ControllerParametersSource=internal  P=1  I=1  UseKiTs=off  D=0  N=100  UseFilter=on  TunerSelectOption=Transfer Function Based (PID Tuner App)  InitialConditionSource=internal  InitialConditionForIntegrator=0  InitialConditionForFilter=0  DifferentiatorICPrevScaledInput=0  ExternalReset=none  TrackingMode=off  Kt=1  LimitOutput=off  SatLimitsSource=internal  UpperSaturationLimit=inf  LowerSaturationLimit=-inf  LinearizeAsGain=off  AntiWindupMode=none  Kb=1  LimitIntegrator=off  UpperIntegratorSaturationLimit=inf  LowerIntegratorSaturationLimit=-inf  POutMin=[]  POutMax=[]  IOutMin=[]  IOutMax=[]  DOutMin=[]  DOutMax=[]  NOutMin=[]  NOutMax=[]  SumOutMin=[]  SumOutMax=[]  SaturationOutMin=[]  SaturationOutMax=[]  PParamMin=[]  PParamMax=[]  IParamMin=[]  IParamMax=[]  DParamMin=[]  DParamMax=[]  NParamMin=[]  NParamMax=[]  KbParamMin=[]  KbParamMax=[]  KtParamMin=[]  KtParamMax=[]  KbOutMin=[]  KbOutMax=[]  KtOutMin=[]  KtOutMax=[]  IntegratorOutMin=[]  IntegratorOutMax=[]  FilterOutMin=[]  FilterOutMax=[]  SumI1OutMin=[]  SumI1OutMax=[]  SumI2OutMin=[]  SumI2OutMax=[]  SumI3OutMin=[]  SumI3OutMax=[]  SumI4OutMin=[]  SumI4OutMax=[]  SumDOutMin=[]  SumDOutMax=[]  DifferentiatorOutMin=[]  DifferentiatorOutMax=[]  FilterDiffOutCoefMin=[]  FilterDiffOutCoefMax=[]  ReciprocalOutMin=[]  ReciprocalOutMax=[]  SumDenOutMin=[]  SumDenOutMax=[]  SumNumOutMin=[]  SumNumOutMax=[]  DivideOutMin=[]  DivideOutMax=[]  UdiffTsProdOutMin=[]  UdiffTsProdOutMax=[]  NTsProdOutMin=[]  NTsProdOutMax=[]  UintegralTsProdOutMin=[]  UintegralTsProdOutMax=[]  UngainTsProdOutMin=[]  UngainTsProdOutMax=[]  ClampingZeroOutDataTypeStr=Inherit: Inherit via back propagation  ClampingZeroOutMin=[]  ClampingZeroOutMax=[]  FilterDenConstantOutDataTypeStr=Inherit: Inherit via back propagation  FilterDenConstantOutMin=[]  FilterDenConstantOutMax=[]  PCopyOutDataTypeStr=Inherit: Inherit via back propagation  PCopyOutMin=[]  PCopyOutMax=[]  NCopyOutDataTypeStr=Inherit: Inherit via back propagation  NCopyOutMin=[]  NCopyOutMax=[]  IntegratorContinuousStateAttributes=''  IntegratorStateMustResolveToSignalObject=off  IntegratorRTWStateStorageClass=Auto  FilterContinuousStateAttributes=''  FilterStateMustResolveToSignalObject=off  FilterRTWStateStorageClass=Auto  ParallelPVariant=InternalParameters  IdealPVariant=Disabled  IVariant=Disabled  DVariant=Disabled  IntegratorVariant=Disabled  SatVariant=Disabled  AWVariant=Disabled  PCopyVariant=Disabled  TRVariant=Disabled  FdbkBlocksVariant=Forward  IdealPFdbkVariant=Disabled  SatFdbkVariant=Disabled  DerivativeFilterVariant=Disabled  NVariant=Disabled  NCopyVariant=Disabled_SignalSpec  FilterICVariant=Disabled  IntegratorICVariant=Disabled  ExternalResetVariant=Disabled  TRSumVariant=Passthrough  SumFdbkVariant=Disabled  SumVariant=Passthrough_P  TsampFilterVariant=InternalTs  TsampNgainVariant=Passthrough  TsampIntegralVariant=Disabled_SignalSpec  ExternalSaturationOutDataTypeStr=Inherit: Same as second input
  Divide{,1..3} (4 alike) : Product  Inputs=***
  Dot Product{,1..5} (6 alike) : DotProduct  OutDataTypeStr=Inherit: Inherit via internal rule
  Gain : Gain  Gain=2/400
  Gain10 : Gain  Gain=2/400
  Ramp{,1..3} (4 alike) : simulink/Sources/Ramp  slope=1  start=0  InitialOutput=0
  Sqrt : Sqrt
  Sum{,1,3,9,18} (5 alike) : Sum  Inputs=|++
  Sum2 : Sum  Inputs=-+|
  u11 : Outport
  Out2 : Outport  Port=2
  wires:
  Constant17/1 -> Divide3/2
  Ramp/1 -> Divide/3
  Sum2/1 -> Dot Product2/1, Dot Product/2
  Divide/1 -> Cos/1
  Cos/1 -> Dot Product/1
  Dot Product/1 -> Gain/1
  Cos1/1 -> Dot Product1/1
  In1/1 -> Delay/1, Sum2/2
  Constant15/1 -> Divide2/2
  Sum18/1 -> Dot Product4/1, Discrete PID Controller1/1, Delay2/1
  [thk] -> Divide3/1
  [thk] -> Divide2/1
  Dot Product4/1 -> Sum9/2
  [thk] -> Divide1/1
  Ramp3/1 -> Divide3/3
  Delay1/1 -> Sum3/2
  Cos2/1 -> Dot Product2/2
  Dot Product2/1 -> Gain10/1
  Cos3/1 -> Dot Product4/2
  Divide2/1 -> Cos2/1
  Constant12/1 -> Divide1/2
  Ramp1/1 -> Divide1/3
  Delay/1 -> Sum2/1
  Sum3/1 -> Discrete PID Controller/1, Dot Product1/2, Delay1/1
  Gain10/1 -> Sum18/1
  Delay2/1 -> Sum18/2
  Constant10/1 -> Divide/2
  Ramp2/1 -> Divide2/3
  Gain/1 -> Sum3/1
  Dot Product1/1 -> Sum9/1
  Sum9/1 -> u11/1
  Constant11/1 -> [thk]
  [thk] -> Divide/1
  Dot Product3/1 -> Add/1
  Dot Product5/1 -> Add/2
  Add/1 -> Sqrt/1
  Sqrt/1 -> Out2/1
  Discrete PID Controller/1 -> Dot Product3/1, Dot Product3/2
  Discrete PID Controller1/1 -> Dot Product5/2, Dot Product5/1
  Divide1/1 -> Sum/1
  Sum/1 -> Cos1/1
  Divide3/1 -> Sum1/1
  Sum1/1 -> Cos3/1
  Constant1/1 -> Sum/2
  Constant2/1 -> Sum1/2

== system xieboduoji_13fangzhennow/node12/PV15kW3/谐波检测/Subsystem/Sub6 ==
  In1 : Inport
  Constant1 : Constant  Value=-60*pi/180
  Constant{10,12,15,17} (4 alike) : Constant  Value=100*pi
  Constant11 : Constant  Value=5
  Constant2 : Constant  Value=-60*pi/180
  Cos : Trigonometry  Operator=cos
  Cos1 : Trigonometry  Operator=cos
  Cos2 : Trigonometry
  Cos3 : Trigonometry
  Delay : Delay  DelayLength=400  SampleTime=5e-5
  Delay1 : Delay  DelayLength=1  SampleTime=5e-5
  Delay2 : Delay  DelayLength=1  SampleTime=5e-5
  Divide{,1..3} (4 alike) : Product  Inputs=***
  Dot Product{,1..2,4} (4 alike) : DotProduct  OutDataTypeStr=Inherit: Inherit via internal rule
  Gain : Gain  Gain=2/400
  Gain10 : Gain  Gain=2/400
  Ramp{,1..3} (4 alike) : simulink/Sources/Ramp  slope=1  start=0  InitialOutput=0
  Sum{,1,3,9,18} (5 alike) : Sum  Inputs=|++
  Sum2 : Sum  Inputs=-+|
  u1 : Outport
  wires:
  [thk] -> Divide/1
  Constant11/1 -> [thk]
  Sum9/1 -> u1/1
  Dot Product1/1 -> Sum9/1
  Gain/1 -> Sum3/1
  Ramp2/1 -> Divide2/3
  Constant10/1 -> Divide/2
  Delay2/1 -> Sum18/2
  Gain10/1 -> Sum18/1
  Sum3/1 -> Delay1/1, Dot Product1/2
  Delay/1 -> Sum2/1
  Ramp1/1 -> Divide1/3
  Constant12/1 -> Divide1/2
  Divide2/1 -> Cos2/1
  Cos3/1 -> Dot Product4/2
  Dot Product2/1 -> Gain10/1
  Cos2/1 -> Dot Product2/2
  Delay1/1 -> Sum3/2
  Ramp3/1 -> Divide3/3
  [thk] -> Divide1/1
  Dot Product4/1 -> Sum9/2
  [thk] -> Divide2/1
  [thk] -> Divide3/1
  Sum18/1 -> Delay2/1, Dot Product4/1
  Constant15/1 -> Divide2/2
  In1/1 -> Sum2/2, Delay/1
  Dot Product/1 -> Gain/1
  Cos/1 -> Dot Product/1
  Divide/1 -> Cos/1
  Sum2/1 -> Dot Product/2, Dot Product2/1
  Ramp/1 -> Divide/3
  Constant17/1 -> Divide3/2
  Cos1/1 -> Dot Product1/1
  Divide1/1 -> Sum/1
  Sum/1 -> Cos1/1
  Sum1/1 -> Cos3/1
  Divide3/1 -> Sum1/1

== system xieboduoji_13fangzhennow/node12/PV15kW3/谐波检测/Subsystem/Sub7 ==
  In1 : Inport
  Constant1 : Constant  Value=-60*pi/180
  Constant{10,12,15,17} (4 alike) : Constant  Value=100*pi
  Constant11 : Constant  Value=7
  Constant2 : Constant  Value=-60*pi/180
  Cos : Trigonometry  Operator=cos
  Cos1 : Trigonometry  Operator=cos
  Cos2 : Trigonometry
  Cos3 : Trigonometry
  Delay : Delay  DelayLength=400  SampleTime=5e-5
  Delay1 : Delay  DelayLength=1  SampleTime=5e-5
  Delay2 : Delay  DelayLength=1  SampleTime=5e-5
  Divide{,1..3} (4 alike) : Product  Inputs=***
  Dot Product{,1..2,4} (4 alike) : DotProduct  OutDataTypeStr=Inherit: Inherit via internal rule
  Gain : Gain  Gain=2/400
  Gain10 : Gain  Gain=2/400
  Ramp{,1..3} (4 alike) : simulink/Sources/Ramp  slope=1  start=0  InitialOutput=0
  Sum{,1,3,9,18} (5 alike) : Sum  Inputs=|++
  Sum2 : Sum  Inputs=-+|
  u1 : Outport
  wires:
  Divide3/1 -> Sum1/1
  Sum1/1 -> Cos3/1
  Sum/1 -> Cos1/1
  Divide1/1 -> Sum/1
  Cos1/1 -> Dot Product1/1
  Constant17/1 -> Divide3/2
  Ramp/1 -> Divide/3
  Sum2/1 -> Dot Product2/1, Dot Product/2
  Divide/1 -> Cos/1
  Cos/1 -> Dot Product/1
  Dot Product/1 -> Gain/1
  In1/1 -> Delay/1, Sum2/2
  Constant15/1 -> Divide2/2
  Sum18/1 -> Dot Product4/1, Delay2/1
  [thk] -> Divide3/1
  [thk] -> Divide2/1
  Dot Product4/1 -> Sum9/2
  [thk] -> Divide1/1
  Ramp3/1 -> Divide3/3
  Delay1/1 -> Sum3/2
  Cos2/1 -> Dot Product2/2
  Dot Product2/1 -> Gain10/1
  Cos3/1 -> Dot Product4/2
  Divide2/1 -> Cos2/1
  Constant12/1 -> Divide1/2
  Ramp1/1 -> Divide1/3
  Delay/1 -> Sum2/1
  Sum3/1 -> Dot Product1/2, Delay1/1
  Gain10/1 -> Sum18/1
  Delay2/1 -> Sum18/2
  Constant10/1 -> Divide/2
  Ramp2/1 -> Divide2/3
  Gain/1 -> Sum3/1
  Dot Product1/1 -> Sum9/1
  Sum9/1 -> u1/1
  Constant11/1 -> [thk]
  [thk] -> Divide/1

== system xieboduoji_13fangzhennow/node12/PV15kW3/谐波检测/Subsystem/Sub8 ==
  In1 : Inport
  Constant1 : Constant  Value=-15*pi/180
  Constant{10,12,15,17} (4 alike) : Constant  Value=100*pi
  Constant11 : Constant  Value=11
  Constant2 : Constant  Value=-15*pi/180
  Cos : Trigonometry  Operator=cos
  Cos2 : Trigonometry
  Cos3 : Trigonometry
  Cos4 : Trigonometry  Operator=cos
  Delay : Delay  DelayLength=400  SampleTime=5e-5
  Delay1 : Delay  DelayLength=1  SampleTime=5e-5
  Delay2 : Delay  DelayLength=1  SampleTime=5e-5
  Divide{,1..3} (4 alike) : Product  Inputs=***
  Dot Product{,1..2,4} (4 alike) : DotProduct  OutDataTypeStr=Inherit: Inherit via internal rule
  Gain : Gain  Gain=2/400
  Gain10 : Gain  Gain=2/400
  Ramp{,1..3} (4 alike) : simulink/Sources/Ramp  slope=1  start=0  InitialOutput=0
  Sum{,1,3,9,18} (5 alike) : Sum  Inputs=|++
  Sum2 : Sum  Inputs=-+|
  u5 : Outport
  wires:
  Sum1/1 -> Cos3/1
  Constant1/1 -> Sum1/2
  Divide3/1 -> Sum1/1
  Cos4/1 -> Dot Product1/1
  Sum/1 -> Cos4/1
  Constant2/1 -> Sum/2
  Divide1/1 -> Sum/1
  Constant17/1 -> Divide3/2
  Ramp/1 -> Divide/3
  Sum2/1 -> Dot Product2/1, Dot Product/2
  Divide/1 -> Cos/1
  Cos/1 -> Dot Product/1
  Dot Product/1 -> Gain/1
  In1/1 -> Delay/1, Sum2/2
  Constant15/1 -> Divide2/2
  Sum18/1 -> Dot Product4/1, Delay2/1
  [thk] -> Divide3/1
  [thk] -> Divide2/1
  Dot Product4/1 -> Sum9/2
  [thk] -> Divide1/1
  Ramp3/1 -> Divide3/3
  Delay1/1 -> Sum3/2
  Cos2/1 -> Dot Product2/2
  Dot Product2/1 -> Gain10/1
  Cos3/1 -> Dot Product4/2
  Divide2/1 -> Cos2/1
  Constant12/1 -> Divide1/2
  Ramp1/1 -> Divide1/3
  Delay/1 -> Sum2/1
  Sum3/1 -> Dot Product1/2, Delay1/1
  Gain10/1 -> Sum18/1
  Delay2/1 -> Sum18/2
  Constant10/1 -> Divide/2
  Ramp2/1 -> Divide2/3
  Gain/1 -> Sum3/1
  Dot Product1/1 -> Sum9/1
  Sum9/1 -> u5/1
  Constant11/1 -> [thk]
  [thk] -> Divide/1

== system xieboduoji_13fangzhennow/node12/PV15kW3/谐波检测/Subsystem/Sub9 ==
  In1 : Inport
  Constant1 : Constant  Value=-15*pi/180
  Constant{10,12,15,17} (4 alike) : Constant  Value=100*pi
  Constant11 : Constant  Value=13
  Constant2 : Constant  Value=-15*pi/180
  Cos : Trigonometry  Operator=cos
  Cos1 : Trigonometry  Operator=cos
  Cos2 : Trigonometry
  Cos3 : Trigonometry
  Delay : Delay  DelayLength=400  SampleTime=5e-5
  Delay1 : Delay  DelayLength=1  SampleTime=5e-5
  Delay2 : Delay  DelayLength=1  SampleTime=5e-5
  Divide{,1..3} (4 alike) : Product  Inputs=***
  Dot Product{,1..2,4} (4 alike) : DotProduct  OutDataTypeStr=Inherit: Inherit via internal rule
  Gain : Gain  Gain=2/400
  Gain10 : Gain  Gain=2/400
  Ramp{,1..3} (4 alike) : simulink/Sources/Ramp  slope=1  start=0  InitialOutput=0
  Sum{,1,3,9,18} (5 alike) : Sum  Inputs=|++
  Sum2 : Sum  Inputs=-+|
  u7 : Outport
  wires:
  Sum1/1 -> Cos3/1
  Constant1/1 -> Sum1/2
  Divide3/1 -> Sum1/1
  Sum/1 -> Cos1/1
  Constant2/1 -> Sum/2
  Divide1/1 -> Sum/1
  [thk] -> Divide/1
  Constant11/1 -> [thk]
  Sum9/1 -> u7/1
  Dot Product1/1 -> Sum9/1
  Gain/1 -> Sum3/1
  Ramp2/1 -> Divide2/3
  Constant10/1 -> Divide/2
  Delay2/1 -> Sum18/2
  Gain10/1 -> Sum18/1
  Sum3/1 -> Delay1/1, Dot Product1/2
  Delay/1 -> Sum2/1
  Ramp1/1 -> Divide1/3
  Constant12/1 -> Divide1/2
  Divide2/1 -> Cos2/1
  Cos3/1 -> Dot Product4/2
  Dot Product2/1 -> Gain10/1
  Cos2/1 -> Dot Product2/2
  Delay1/1 -> Sum3/2
  Ramp3/1 -> Divide3/3
  [thk] -> Divide1/1
  Dot Product4/1 -> Sum9/2
  [thk] -> Divide2/1
  [thk] -> Divide3/1
  Sum18/1 -> Delay2/1, Dot Product4/1
  Constant15/1 -> Divide2/2
  In1/1 -> Sum2/2, Delay/1
  Cos1/1 -> Dot Product1/1
  Dot Product/1 -> Gain/1
  Cos/1 -> Dot Product/1
  Divide/1 -> Cos/1
  Sum2/1 -> Dot Product/2, Dot Product2/1
  Ramp/1 -> Divide/3
  Constant17/1 -> Divide3/2

== system xieboduoji_13fangzhennow/node12/PV15kW3/谐波检测/Subsystem/Subsystem2 ==
  u1 : Inport
  u2 : Inport  Port=2
  u3 : Inport  Port=3
  u4 : Inport  Port=4
  u5 : Inport  Port=5
  u6 : Inport  Port=6
  u7 : Inport  Port=7
  u8 : Inport  Port=8
  u9 : Inport  Port=9
  u10 : Inport  Port=10
  u11 : Inport  Port=11
  u12 : Inport  Port=12
  Pul : DiscretePulseGenerator  PulseType=Time based  Period=5e-5  PulseWidth=40
  RMS1 : Subsystem  TreatAsAtomicUnit=on
  k1 : Outport  VectorParamsAs1DForOutWhenUnconnected=off
  k2 : Outport  Port=2  VectorParamsAs1DForOutWhenUnconnected=off
  k3 : Outport  Port=3  VectorParamsAs1DForOutWhenUnconnected=off
  k4 : Outport  Port=4  VectorParamsAs1DForOutWhenUnconnected=off
  k5 : Outport  Port=5  VectorParamsAs1DForOutWhenUnconnected=off
  k6 : Outport  Port=6  VectorParamsAs1DForOutWhenUnconnected=off
  wires:
  Pul/1 -> RMS1/Trigger
  u1/1 -> RMS1/1(u1)
  u2/1 -> RMS1/2(i1)
  u3/1 -> RMS1/3(u3)
  u4/1 -> RMS1/4(u4)
  u5/1 -> RMS1/5(u5)
  u6/1 -> RMS1/6(u6)
  RMS1/2(k2) -> k2/1
  RMS1/3(k3) -> k3/1
  RMS1/4(k4) -> k4/1
  RMS1/1(k1) -> k1/1
  RMS1/6(k6) -> k6/1
  RMS1/5(k5) -> k5/1
  u12/1 -> RMS1/12(u10)
  u11/1 -> RMS1/11(u9)
  u10/1 -> RMS1/10(u8)
  u9/1 -> RMS1/9(u7)
  u8/1 -> RMS1/8(i2)
  u7/1 -> RMS1/7(u2)

== system xieboduoji_13fangzhennow/node12/PV15kW3/谐波检测/Subsystem2/RMS1 ==
  u1 : Inport
  i1 : Inport  Port=2
  u3 : Inport  Port=3
  u4 : Inport  Port=4
  u5 : Inport  Port=5
  u6 : Inport  Port=6
  u2 : Inport  Port=7
  i2 : Inport  Port=8
  u7 : Inport  Port=9
  u8 : Inport  Port=10
  u9 : Inport  Port=11
  u10 : Inport  Port=12
  Trigger : TriggerPort  VariantControl=(inherit)
  Scope : Scope
  xunidiandao : MATLAB Function  TreatAsAtomicUnit=on
  k1 : Outport  VectorParamsAs1DForOutWhenUnconnected=off
  k2 : Outport  Port=2  VectorParamsAs1DForOutWhenUnconnected=off
  k3 : Outport  Port=3  VectorParamsAs1DForOutWhenUnconnected=off
  k4 : Outport  Port=4  VectorParamsAs1DForOutWhenUnconnected=off
  k5 : Outport  Port=5  VectorParamsAs1DForOutWhenUnconnected=off
  k6 : Outport  Port=6  VectorParamsAs1DForOutWhenUnconnected=off
  wires:
  xunidiandao/1(k1) -> k1/1
  u1/1 -> xunidiandao/1(u1)
  xunidiandao/2(k2) -> k2/1
  xunidiandao/3(k3) -> k3/1
  xunidiandao/4(k4) -> k4/1
  xunidiandao/5(k5) -> k5/1
  xunidiandao/6(k6) -> k6/1
  i1/1 -> xunidiandao/2(i1)
  u3/1 -> xunidiandao/3(u2)
  u4/1 -> xunidiandao/4(i2)
  u5/1 -> xunidiandao/5(u3)
  u6/1 -> xunidiandao/6(i3)
  u10/1 -> xunidiandao/12(i6)
  u9/1 -> xunidiandao/11(u6)
  u8/1 -> xunidiandao/10(i5)
  u7/1 -> xunidiandao/9(u5)
  i2/1 -> xunidiandao/8(i4)
  u2/1 -> xunidiandao/7(u4)
  xunidiandao/7(k0) -> Scope/1

== system xieboduoji_13fangzhennow/node14/PV15kW3/谐波检测/DFT6-24A3/Sub ==
  In1 : Inport
  Constant{10,12,15,17} (4 alike) : Constant  Value=100*pi
  Constant11 : Constant  Value=5
  Cos : Trigonometry  Operator=cos
  Cos1 : Trigonometry  Operator=cos
  Cos2 : Trigonometry
  Cos3 : Trigonometry
  Delay : Delay  DelayLength=400  SampleTime=5e-5
  Delay1 : Delay  DelayLength=1  SampleTime=5e-5
  Delay2 : Delay  DelayLength=1  SampleTime=5e-5
  Divide{,1..3} (4 alike) : Product  Inputs=***
  Dot Product{,1..2,4} (4 alike) : DotProduct  OutDataTypeStr=Inherit: Inherit via internal rule
  Gain : Gain  Gain=2/400
  Gain10 : Gain  Gain=2/400
  Ramp{,1..3} (4 alike) : simulink/Sources/Ramp  slope=1  start=0  InitialOutput=0
  Sum18 : Sum  Inputs=|++
  Sum2 : Sum  Inputs=-+|
  Sum3 : Sum  Inputs=|++
  Sum9 : Sum  Inputs=|++
  Out1 : Outport
  wires:
  Constant17/1 -> Divide3/2
  Ramp/1 -> Divide/3
  Sum2/1 -> Dot Product2/1, Dot Product/2
  Divide/1 -> Cos/1
  Cos/1 -> Dot Product/1
  Dot Product/1 -> Gain/1
  Cos1/1 -> Dot Product1/1
  In1/1 -> Delay/1, Sum2/2
  Constant15/1 -> Divide2/2
  Sum18/1 -> Dot Product4/1, Delay2/1
  [thk] -> Divide3/1
  [thk] -> Divide2/1
  Dot Product4/1 -> Sum9/2
  [thk] -> Divide1/1
  Ramp3/1 -> Divide3/3
  Divide3/1 -> Cos3/1
  Delay1/1 -> Sum3/2
  Cos2/1 -> Dot Product2/2
  Dot Product2/1 -> Gain10/1
  Cos3/1 -> Dot Product4/2
  Divide2/1 -> Cos2/1
  Constant12/1 -> Divide1/2
  Ramp1/1 -> Divide1/3
  Divide1/1 -> Cos1/1
  Delay/1 -> Sum2/1
  Sum3/1 -> Dot Product1/2, Delay1/1
  Gain10/1 -> Sum18/1
  Delay2/1 -> Sum18/2
  Constant10/1 -> Divide/2
  Ramp2/1 -> Divide2/3
  Gain/1 -> Sum3/1
  Dot Product1/1 -> Sum9/1
  Sum9/1 -> Out1/1
  Constant11/1 -> [thk]
  [thk] -> Divide/1

== system xieboduoji_13fangzhennow/node14/PV15kW3/谐波检测/DFT6-24A3/Sub1 ==
  In1 : Inport
  Constant{10,12,15,17} (4 alike) : Constant  Value=100*pi
  Constant11 : Constant  Value=7
  Cos : Trigonometry  Operator=cos
  Cos1 : Trigonometry  Operator=cos
  Cos2 : Trigonometry
  Cos3 : Trigonometry
  Delay : Delay  DelayLength=400  SampleTime=5e-5
  Delay1 : Delay  DelayLength=1  SampleTime=5e-5
  Delay2 : Delay  DelayLength=1  SampleTime=5e-5
  Divide{,1..3} (4 alike) : Product  Inputs=***
  Dot Product{,1..2,4} (4 alike) : DotProduct  OutDataTypeStr=Inherit: Inherit via internal rule
  Gain : Gain  Gain=2/400
  Gain10 : Gain  Gain=2/400
  Ramp{,1..3} (4 alike) : simulink/Sources/Ramp  slope=1  start=0  InitialOutput=0
  Sum18 : Sum  Inputs=|++
  Sum2 : Sum  Inputs=-+|
  Sum3 : Sum  Inputs=|++
  Sum9 : Sum  Inputs=|++
  Out1 : Outport
  wires:
  [thk] -> Divide/1
  Constant11/1 -> [thk]
  Sum9/1 -> Out1/1
  Dot Product1/1 -> Sum9/1
  Gain/1 -> Sum3/1
  Ramp2/1 -> Divide2/3
  Constant10/1 -> Divide/2
  Delay2/1 -> Sum18/2
  Gain10/1 -> Sum18/1
  Sum3/1 -> Delay1/1, Dot Product1/2
  Delay/1 -> Sum2/1
  Divide1/1 -> Cos1/1
  Ramp1/1 -> Divide1/3
  Constant12/1 -> Divide1/2
  Divide2/1 -> Cos2/1
  Cos3/1 -> Dot Product4/2
  Dot Product2/1 -> Gain10/1
  Cos2/1 -> Dot Product2/2
  Delay1/1 -> Sum3/2
  Divide3/1 -> Cos3/1
  Ramp3/1 -> Divide3/3
  [thk] -> Divide1/1
  Dot Product4/1 -> Sum9/2
  [thk] -> Divide2/1
  [thk] -> Divide3/1
  Sum18/1 -> Delay2/1, Dot Product4/1
  Constant15/1 -> Divide2/2
  In1/1 -> Sum2/2, Delay/1
  Cos1/1 -> Dot Product1/1
  Dot Product/1 -> Gain/1
  Cos/1 -> Dot Product/1
  Divide/1 -> Cos/1
  Sum2/1 -> Dot Product/2, Dot Product2/1
  Ramp/1 -> Divide/3
  Constant17/1 -> Divide3/2
